simulink model "calibration_pumps"  (R2026a)
settings: Solver=VariableStepAuto  StopTime=inf
InitFcn:
  | coefficients = [0,coefficients];
StopFcn:
  | Q = out.Q;
  | save(fullfile('calibration_data','pump_calibration.mat'),'Q');
settings Model: Creator=user  LastModifiedBy=user

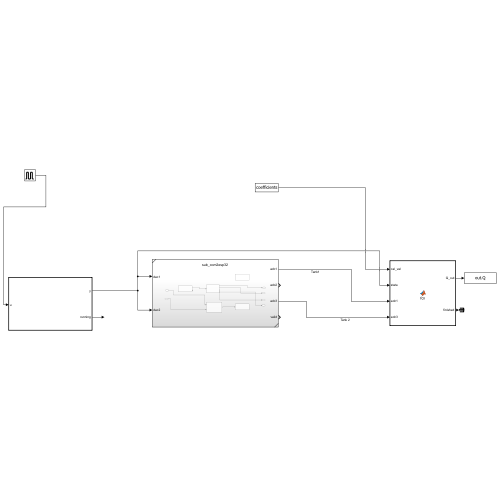
[thumbnail: Simulink's stored preview of the top-level diagram]
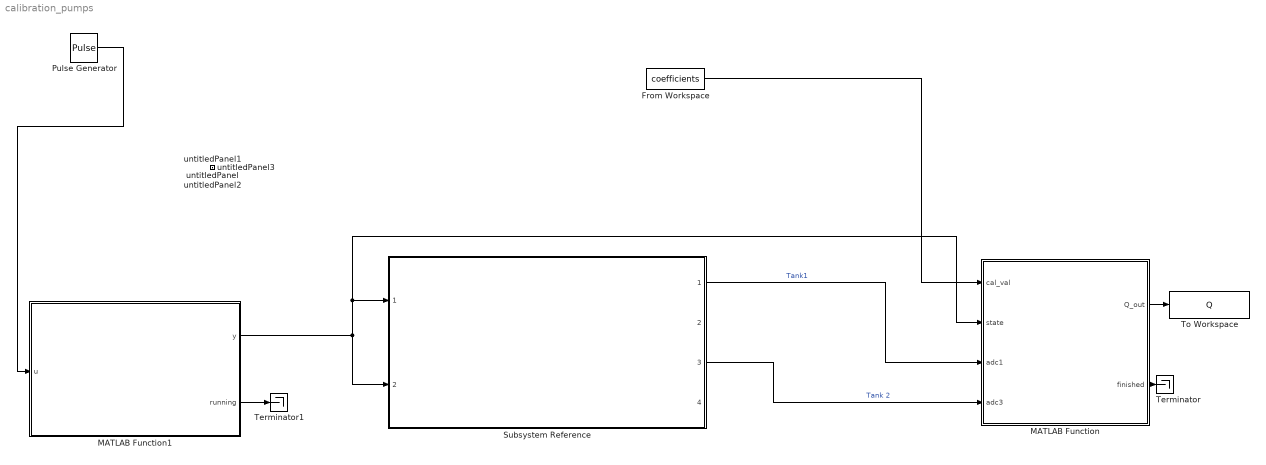
== system calibration_pumps ==
  From Workspace : FromWorkspace  VariableName=coefficients  SampleTime=-1
  MATLAB Function : MATLAB Function  TreatAsAtomicUnit=on
  MATLAB Function1 : MATLAB Function  TreatAsAtomicUnit=on
  Pulse Generator : DiscretePulseGenerator  PulseType=Time based  Period=12  PulseWidth=20
  Subsystem Reference : Subsystem  ReferencedSubsystem=sub_com2esp32
  Terminator : Terminator
  Terminator1 : Terminator
  To Workspace : ToWorkspace  VariableName=Q  SampleTime=-1
      settings: MaxDataPoints=1
  untitledPanel : Subsystem  Tag=HiddenForWebPanel  IsWebBlockPanel=on
  untitledPanel1 : Subsystem  Tag=HiddenForWebPanel  IsWebBlockPanel=on
  untitledPanel2 : Subsystem  Tag=HiddenForWebPanel  IsWebBlockPanel=on
  untitledPanel3 : Subsystem  Tag=HiddenForWebPanel  IsWebBlockPanel=on
  wires:
  Subsystem Reference/3 -> MATLAB Function/4(adc3)  "Tank 2"
  Subsystem Reference/1 -> MATLAB Function/3(adc1)  "Tank1"
  MATLAB Function/1(Q_out) -> To Workspace/1
  MATLAB Function/2(finished) -> Terminator/1
  MATLAB Function1/1(y) -> MATLAB Function/2(state), Subsystem Reference/1, Subsystem Reference/2
  From Workspace/1 -> MATLAB Function/1(cal_val)
  Pulse Generator/1 -> MATLAB Function1/1(u)
  MATLAB Function1/2(running) -> Terminator1/1

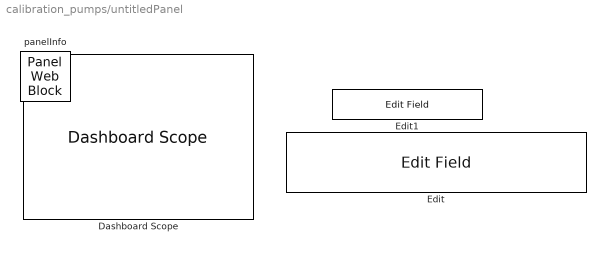
== system calibration_pumps/untitledPanel ==
  Dashboard Scope : DashboardScope  Tag=HiddenForWebPanel  PanelInfo="{\"height\":195,\"left\":22,\"panelId\":\"panelId-0a8f6d05-5e0e-4052-8464-4cdde78ccbfe\",\"top\":22,\"type\":\"panelChild\",\"version\":\"2019b\",\"width\":271,\"zIndex\":1500002}"  FontColor=[0.0, 0.0, 0.0]
  Edit : EditField  Tag=HiddenForWebPanel  PanelInfo="{\"height\":25,\"left\":322,\"panelId\":\"panelId-0a8f6d05-5e0e-4052-8464-4cdde78ccbfe\",\"top\":100,\"type\":\"panelChild\",\"version\":\"2019b\",\"width\":181,\"zIndex\":1500006}"  LabelPosition=Hide  ShowInitialText=on  Alignment=Center
  Edit1 : EditField  Tag=HiddenForWebPanel  PanelInfo="{\"height\":30,\"left\":327,\"panelId\":\"panelId-0a8f6d05-5e0e-4052-8464-4cdde78ccbfe\",\"top\":53,\"type\":\"panelChild\",\"version\":\"2019b\",\"width\":150,\"zIndex\":1500004}"  LabelPosition=Hide  ShowInitialText=on  Alignment=Center
  panelInfo : PanelWebBlock  Tag=HiddenForWebPanel  PanelInfo="{\"compacted\":false,\"height\":362,\"isActiveTab\":false,\"left\":183,\"name\":\"Panel\",\"panelId\":\"panelId-0a8f6d05-5e0e-4052-8464-4cdde78ccbfe\",\"popoutData\":{\"height\":495,\"left\":546,\"maximized\":false,\"top\":827,\"width\":618},\"popoutMode\":\"windowHidden\",\"tabIndex\":0,\"tabbedSetId\":\"tabbedSet4972758365\",\"top\":737,\"type\":\"panel\",\"version\":\"2019b\",\"visible\":false,\"width\":602,\"zIndex\":1500002}"  PanelSnapshot=<binary blob, 20028 chars, not shown>

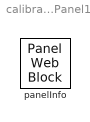
== system calibration_pumps/untitledPanel1 ==
  panelInfo : PanelWebBlock  Tag=HiddenForWebPanel  PanelInfo="{\"compacted\":false,\"height\":362,\"isActiveTab\":true,\"left\":183,\"name\":\"Panel1\",\"panelId\":\"panelId-b2ee2f41-7720-49f1-b51a-3062c351f597\",\"popoutData\":{\"height\":495,\"left\":546,\"maximized\":false,\"top\":827,\"width\":618},\"popoutMode\":\"windowHidden\",\"tabIndex\":1,\"tabbedSetId\":\"tabbedSet4972758365\",\"top\":737,\"type\":\"panel\",\"version\":\"2019b\",\"visible\":true,\"width\":602,\"zIndex\":1500004}"

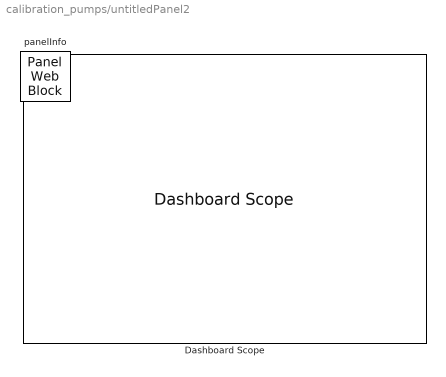
== system calibration_pumps/untitledPanel2 ==
  Dashboard Scope : DashboardScope  Tag=HiddenForWebPanel  PanelInfo="{\"height\":289,\"left\":18,\"panelId\":\"panelId-8ba459e9-7eb9-43d1-9a8b-2b7bff5a2d5c\",\"top\":18,\"type\":\"panelChild\",\"version\":\"2019b\",\"width\":403,\"zIndex\":1500002}"  FontColor=[0.0, 0.0, 0.0]
  panelInfo : PanelWebBlock  Tag=HiddenForWebPanel  PanelInfo="{\"compacted\":false,\"height\":329,\"isActiveTab\":true,\"left\":1320,\"name\":\"Panel2\",\"panelId\":\"panelId-8ba459e9-7eb9-43d1-9a8b-2b7bff5a2d5c\",\"popoutData\":{\"height\":440,\"left\":1683,\"maximized\":false,\"top\":822,\"width\":459},\"popoutMode\":\"windowHidden\",\"tabIndex\":0,\"tabbedSetId\":\"tabbedSet1724704130\",\"top\":710,\"type\":\"panel\",\"version\":\"2019b\",\"visible\":true,\"width\":443,\"zIndex\":1500006}"  PanelSnapshot=<binary blob, 75208 chars, not shown>

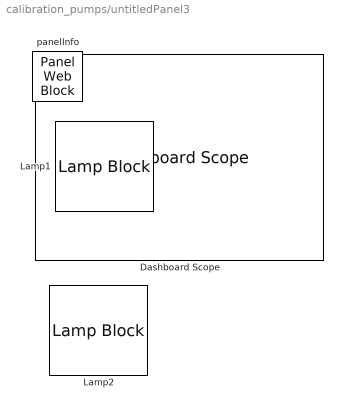
== system calibration_pumps/untitledPanel3 ==
  Dashboard Scope : DashboardScope  Tag=HiddenForWebPanel  PanelInfo="{\"height\":401,\"left\":232,\"panelId\":\"panelId-037cc253-1a0e-430c-bfc3-d197bdfa8fb6\",\"top\":22,\"type\":\"panelChild\",\"version\":\"2019b\",\"width\":585,\"zIndex\":1500002}"  FontColor=[0.0, 0.0, 0.0]
  Lamp1 : LampBlock  Tag=HiddenForWebPanel  PanelInfo="{\"height\":90,\"left\":31,\"panelId\":\"panelId-037cc253-1a0e-430c-bfc3-d197bdfa8fb6\",\"top\":87,\"type\":\"panelChild\",\"version\":\"2019b\",\"width\":98,\"zIndex\":1500004}"  LabelPosition=Hide  DefaultColor=[192.0, 192.0, 192.0]
  Lamp2 : LampBlock  Tag=HiddenForWebPanel  PanelInfo="{\"height\":90,\"left\":32,\"panelId\":\"panelId-037cc253-1a0e-430c-bfc3-d197bdfa8fb6\",\"top\":249,\"type\":\"panelChild\",\"version\":\"2019b\",\"width\":98,\"zIndex\":1500006}"  LabelPosition=Hide  DefaultColor=[192.0, 192.0, 192.0]
  panelInfo : PanelWebBlock  Tag=HiddenForWebPanel  PanelInfo="{\"compacted\":false,\"height\":453,\"isActiveTab\":true,\"labels\":{\"label0415151059\":{\"deleted\":false,\"left\":32,\"settings\":{\"backgroundColor\":\"rgba(0, 0, 0, 0)\",\"bold\":true,\"font\":\"Arial\",\"fontColor\":\"black\",\"fontSize\":1.2000000000000002,\"italicized\":false,\"underlined\":false},\"text\":\"Pump\",\"top\":59},\"label6487320007\":{\"deleted\":false,\"left\":29,\"settings\":{\"backgroundColor\":\"rgba(0, 0, 0, 0)\",\"bold\":true,\"font\":\"Arial\",\"fontColor\":\"black\",\"fontSize\":1.1,\"italicized\":false,\"underlined\":false},\"text\":\"Calibration finished\",\"top\":221}},\"left\":205,\"name\":\"Panel3\",\"panelId\":\"panelId-037cc253-1a0e-430c-bfc3-d197bdfa8fb6\",\"tabIndex\":0,\"tabbedSetId\":\"tabbedSet3591606152\",\"top\":32,\"type\":\"panel\",\"version\":\"2019b\",\"visible\":true,\"width\":837,\"zIndex\":1500008}"  PanelSnapshot=<binary blob, 54716 chars, not shown>

== matlab function calibration_pumps/MATLAB Function ==
  data: Q_out output; finished output; cal_val input; state input; adc1 input; adc3 input
function [Q_out,finished] = fcn(cal_val, state, adc1, adc3)

persistent sensor_low sensor_high prev_state Q counter cal

if isempty(sensor_low) && isempty(sensor_high)
    sensor_low = zeros(2,1);
    sensor_high = zeros(2,1);
    counter = 0;

    % 改成 2x9，第一列留给 DAC=255 -> Q=0
    Q = zeros(2,9);

    prev_state = 255;
    cal = [cal_val(1); cal_val(3)];
end

A = 154;
dt = 12 * 0.8;

% 进入新的 LOW 阶段时，计算上一个 LOW 阶段的流量
if state ~= 255 && prev_state == 255 && counter > 0 && counter < 8
    sensor_high = [adc1; adc3] .* cal * A;

    % counter=1 对应 DAC=223，存到 Q(:,2)
    % counter=2 对应 DAC=191，存到 Q(:,3)
    Q(:, counter + 1) = (sensor_high - sensor_low) / dt;
end

% 新 LOW 阶段开始，记录初始液位
if state ~= 255 && prev_state == 255
    sensor_low = [adc1; adc3] .* cal * A;
    counter = counter + 1;
end

% 最后一个 LOW 阶段结束，计算 DAC=0 的流量
if counter == 8 && state == 255
    sensor_high = [adc1; adc3] .* cal * A;

    % counter=8 对应 DAC=0，存到 Q(:,9)
    Q(:,9) = (sensor_high - sensor_low) / dt;

    finished = 1;
    counter = counter + 1;

elseif counter > 8
    finished = 1;
else
    finished = 0;
end

prev_state = state;
Q_out = Q;

end

== matlab function calibration_pumps/MATLAB Function1 ==
  data: u input; y output; running output
function [y,running] = fcn(u)
persistent counter2 prev_u

if isempty(counter2) && isempty(prev_u)
    counter2 =0; 
    prev_u =0; 
end
running = 1;

if u ==1 && prev_u ==0
    counter2 = counter2 +1;
end
if u ==0
    s = 0.125 * counter2; 
    if s <= 1
        y = 255 * (1-s);
        running =0;
    else 
        y = 255; 
    end
else
    y = 255; 
end

prev_u = u;
